simulink model "sys_2"  (R2017a)
settings: Solver=FixedStepAuto  StartTime=0.0  StopTime=40  FixedStep=0.02  RelTol=1e-3
values from neighbouring files (symbols this model uses):
  D = zeros(1,1)    [OBS_CONT.m]
  F = [0 1 0 0;-k/j2 -b/j2 k/j2 b/j2;0 0 0 01;k/j1 b/j1 -k/j1 -b/j1]    [OBS_CONT.m]
  G = [0;0;0;1/j1]    [OBS_CONT.m]
  H = [1 0 0 0]    [OBS_CONT.m]
  Kc = [-0.26139 0.041515 0.65538 1.1604]    [OBS_CONT.m]
  Ke = [22.0004 242.0531 1512.84032 5485.9822]'    [OBS_CONT.m]
settings Model: Creator=ASUS  LastModifiedBy=ASUS

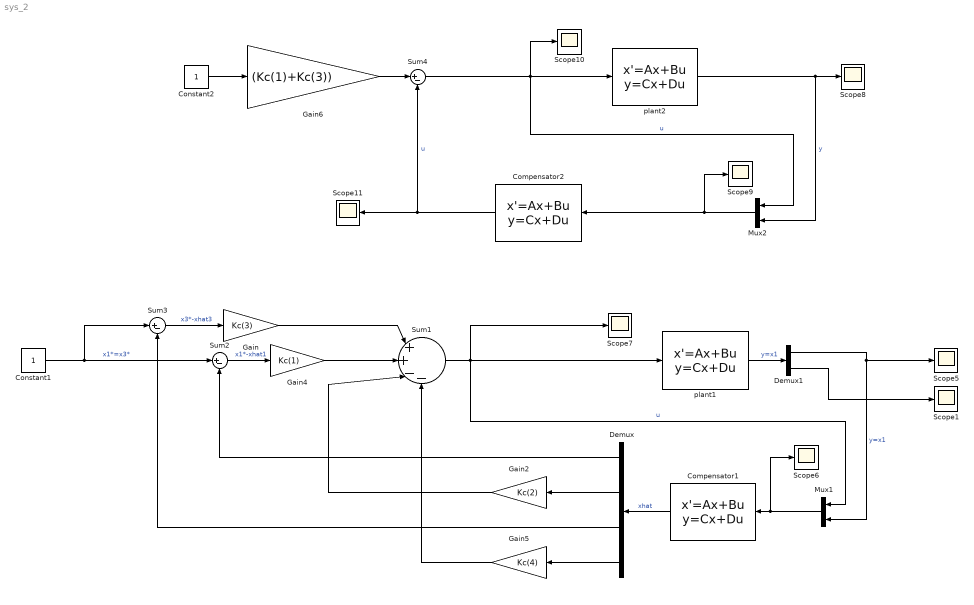
== system sys_2 ==
  Compensator1 : StateSpace  A=F-Ke*H  B=[G Ke]  C=[1 0 0 0;0 1 0 0;0 0 1 0;0 0 0 1]  D=[0 0;0 0;0 0;0 0]  X0=0
  Compensator2 : StateSpace  A=F-Ke*H  B=[G Ke]  C=Kc  D=[D D]  X0=0
  Constant1 : Constant
  Constant2 : Constant
  Demux : Demux
  Demux1 : Demux  Outputs=2
  Gain : Gain  Gain=Kc(3)
  Gain2 : Gain  Gain=Kc(2)
  Gain4 : Gain  Gain=Kc(1)
  Gain5 : Gain  Gain=Kc(4)
  Gain6 : Gain  Gain=(Kc(1)+Kc(3))
  Mux1 : Mux  Inputs=2
  Mux2 : Mux  Inputs=2
  Scope{1,5..11} (8 alike) : Scope
  Sum1 : Sum  Inputs=|++--
  Sum2 : Sum  Inputs=|+-
  Sum3 : Sum  Inputs=|+-
  Sum4 : Sum  Inputs=|+-
  plant1 : StateSpace  A=F  B=G  C=[1 0 0 0;0 0 1 0]  D=[0;0]  X0=0
  plant2 : StateSpace  A=F  B=G  C=H  D=D  X0=0
  wires:
  Mux1/1 -> Scope6/1, Compensator1/1
  Sum1/1 -> Scope7/1, plant1/1, Mux1/1  "u"
  Demux1/1 -> Mux1/2, Scope5/1  "y=x1"
  Compensator1/1 -> Demux/1  "xhat"
  Demux/1 -> Sum2/2
  Gain2/1 -> Sum1/3
  Demux/3 -> Sum3/2
  Demux/2 -> Gain2/1
  Gain4/1 -> Sum1/2
  Sum2/1 -> Gain4/1  "x1*-xhat1"
  Constant1/1 -> Sum3/1, Sum2/1  "x1*=x3*"
  Sum3/1 -> Gain/1  "x3*-xhat3"
  Demux/4 -> Gain5/1
  Gain/1 -> Sum1/1
  Constant2/1 -> Gain6/1
  Sum4/1 -> Scope10/1, Mux2/1, plant2/1  "u"
  plant2/1 -> Mux2/2, Scope8/1  "y"
  Mux2/1 -> Scope9/1, Compensator2/1
  Compensator2/1 -> Sum4/2, Scope11/1  "u"
  Gain6/1 -> Sum4/1
  Gain5/1 -> Sum1/4
  plant1/1 -> Demux1/1  "y=x1"
  Demux1/2 -> Scope1/1
